simulink model "Priklad_2"  (R2022b)
settings: Solver=VariableStepAuto  StartTime=0.0  StopTime=150  RelTol=1e-3
settings Model: Creator=honza  LastModifiedBy=honza

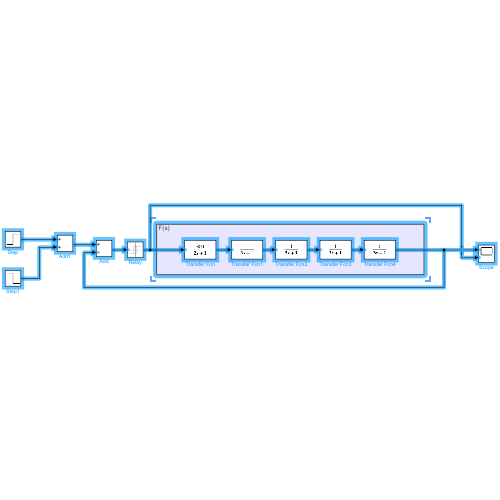
[thumbnail: Simulink's stored preview of the top-level diagram]
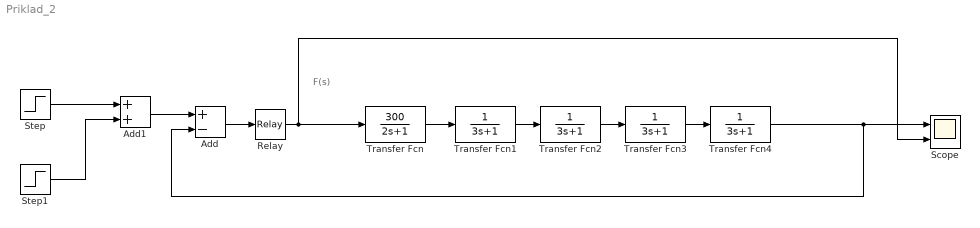
== system Priklad_2 ==
  note: F(s)
  Add : Sum  Inputs=+-
  Add1 : Sum
  Relay : Relay  OnSwitchValue=1  OffSwitchValue=-1
  Scope : Scope  NumInputPorts=2
  Step : Step  Time=0  After=250  SampleTime=0
  Step1 : Step  Time=100  Before=250  After=180  SampleTime=0
  Transfer Fcn : TransferFcn  Numerator=[300]  Denominator=[2 1]
  Transfer Fcn{1..4} (4 alike) : TransferFcn  Denominator=[3 1]
  wires:
  Transfer Fcn1/1 -> Transfer Fcn2/1
  Transfer Fcn2/1 -> Transfer Fcn3/1
  Transfer Fcn3/1 -> Transfer Fcn4/1
  Transfer Fcn/1 -> Transfer Fcn1/1
  Relay/1 -> Transfer Fcn/1, Scope/2
  Add/1 -> Relay/1
  Transfer Fcn4/1 -> Add/2, Scope/1
  Add1/1 -> Add/1
  Step/1 -> Add1/1
  Step1/1 -> Add1/2
